simulink model "Copy_of_CDPR"  (R2023b)
settings: Solver=FixedStepDiscrete  StartTime=0.0  StopTime=10  FixedStep=0.001  RelTol=1e-3
values from neighbouring files (symbols this model uses):
  qi = R\l0    [Initialisation.m]
  R = (sqrt(0.08^2 + 0.005^2/(2*pi))/25)    [DynModel_q.m]    (also in Initialisation.m = (sqrt(0.08^2 + 0.005^2/(2*pi))/25)   * eye(8); Rot.m = Rz * Ry * Rx; Rz.m = [cos(theta) -sin(theta) 0)
  tau_ci = quadprog(H, f, [], [], Aeq, beq, 50*ones(8,1), 5000*ones(8,1))    [Initialisation.m]    (also in TDA.m = u(13:20))
  Xi = [0, 0.0, 2.2, 0, 0, 0]'    [Initialisation.m]
libraries: simulink x2
settings Model: Creator=abellila  LastModifiedBy=abellila
settings SolverCC: SolverJacobianMethodControl=FullAnalytical

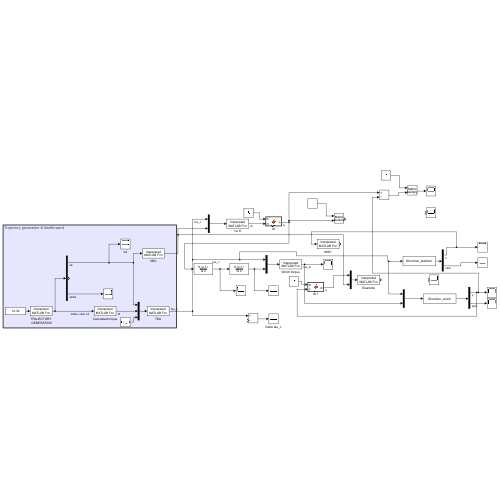
[thumbnail: Simulink's stored preview of the top-level diagram]
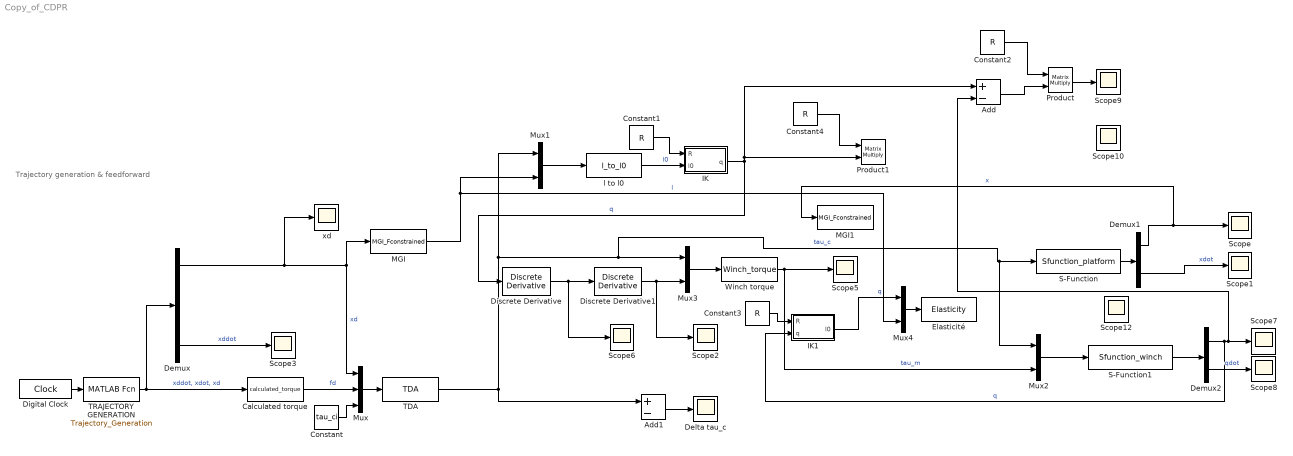
== system Copy_of_CDPR ==
  note: Trajectory generation & feedforward
  Add : Sum  Inputs=+-
  Add1 : Sum  Inputs=+-
  Calculated torque : MATLABFcn  MATLABFcn=calculated_torque  Output1D=off
  Constant : Constant  Value=tau_ci
  Constant{1..4} (4 alike) : Constant  Value=R
  Delta tau_c : Scope
  Demux : Demux  Outputs=3
  Demux1 : Demux  Outputs=2
  Demux2 : Demux  Outputs=2
  Digital Clock : DigitalClock  SampleTime=0.001
  Discrete Derivative : simulink/Discrete/Discrete Derivative  gainval=1.0  ICPrevScaledInput=0.0  OutMin=[]  OutMax=[]  OutDataType=fixdt(1, 16)  OutScaling=2^-10  DoSatur=off
  Discrete Derivative1 : simulink/Discrete/Discrete Derivative  gainval=1.0  ICPrevScaledInput=0.0  OutMin=[]  OutMax=[]  OutDataType=fixdt(1, 16)  OutScaling=2^-10  DoSatur=off
  Elasticité : MATLABFcn  MATLABFcn=Elasticity  OutputDimensions=8  Output1D=off
  IK : MATLAB Function  TreatAsAtomicUnit=on
  IK1 : MATLAB Function  TreatAsAtomicUnit=on
  MGI : MATLABFcn  MATLABFcn=MGI_Fconstrained
  MGI1 : MATLABFcn  MATLABFcn=MGI_Fconstrained  OutputDimensions=8  Output1D=off
  Mux : Mux  Inputs=3
  Mux{1..4} (4 alike) : Mux  Inputs=2
  Product : Product  Multiplication=Matrix(*)
  Product1 : Product  Multiplication=Matrix(*)
  S-Function : S-Function  FunctionName=Sfunction_platform  Parameters=[Xi;zeros(6,1)]  SFunctionDeploymentMode=off  EnableBusSupport=off
  S-Function1 : S-Function  FunctionName=Sfunction_winch  Parameters=[qi;zeros(8,1)]  SFunctionDeploymentMode=off  EnableBusSupport=off
  Scope{,1..3,5..10,12} (11 alike) : Scope
  TDA : MATLABFcn  MATLABFcn=TDA  OutputDimensions=8  Output1D=off
  TRAJECTORY GENERATION : MATLABFcn  MATLABFcn=Trajectory_Generation  Output1D=off
  Winch torque : MATLABFcn  MATLABFcn=Winch_torque
  l to l0 : MATLABFcn  MATLABFcn=l_to_l0  OutputDimensions=8  OutputSignalType=real  Output1D=off
  xd : Scope
  wires:
  Digital Clock/1 -> TRAJECTORY GENERATION/1
  TRAJECTORY GENERATION/1 -> Calculated torque/1, Demux/1  "xddot, xdot, xd"
  Demux/1 -> MGI/1, Mux/1, xd/1  "xd"
  Mux/1 -> TDA/1
  TDA/1 -> Add1/1, Mux1/1, Mux2/1, S-Function/1, Mux3/1  "tau_c"
  S-Function/1 -> Demux1/1
  Demux1/1 -> MGI1/1, Scope/1  "x"
  Demux1/2 -> Scope1/1  "xdot"
  Constant/1 -> Mux/3
  Calculated torque/1 -> Mux/2  "fd"
  Demux/3 -> Scope3/1  "xddot"
  MGI/1 -> Mux4/2, Mux1/2  "l"
  Mux1/1 -> l to l0/1
  Mux3/1 -> Winch torque/1
  IK/1(q) -> Discrete Derivative/1, Product1/2, Add/1  "q"
  Discrete Derivative/1 -> Discrete Derivative1/1, Scope6/1
  l to l0/1 -> IK/2(l0)  "l0"
  Constant1/1 -> IK/1(R)
  Discrete Derivative1/1 -> Scope2/1, Mux3/2
  Winch torque/1 -> Scope5/1, Mux2/2  "tau_m"
  Mux2/1 -> S-Function1/1
  Demux2/1 -> IK1/2(q), Add/2, Scope7/1  "q"
  Demux2/2 -> Scope8/1  "qdot"
  S-Function1/1 -> Demux2/1
  Mux4/1 -> Elasticité/1
  Constant2/1 -> Product/1
  Add/1 -> Product/2
  Product/1 -> Scope9/1
  Add1/1 -> Delta tau_c/1
  Constant3/1 -> IK1/1(R)
  Constant4/1 -> Product1/1
  IK1/1(l0) -> Mux4/1  "q"

== matlab function Copy_of_CDPR/IK ==
  data: R input; q output; l0 input
function q = fcn(R, l0)

q = R\l0;

== matlab function Copy_of_CDPR/IK1 ==
  data: R input; l0 output; q input
function l0 = fcn(R, q)

l0 = R*q;
